simulink model "motor_cont_ctrl0"  (R2018a)
settings: Solver=FixedStepAuto  StartTime=0.0  StopTime=30  RelTol=1e-3
libraries: simulink x1
settings Model: Creator=HuuNgan  LastModifiedBy=HuuNgan

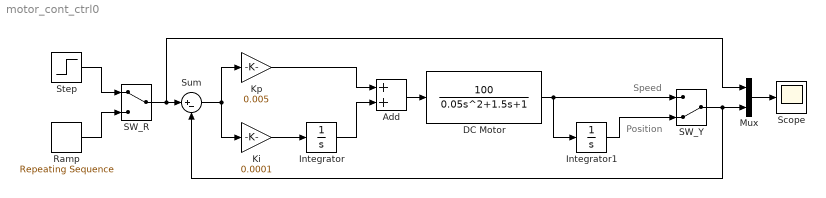
== system motor_cont_ctrl0 ==
  note: Position
  note: Speed
  Add : Sum
  DC Motor : TransferFcn  Numerator=[100]  Denominator=[0.05 1.5 1]
  "Integrator " : Integrator
  Integrator1 : Integrator
  Ki : Gain  Gain=0.0001
  Kp : Gain  Gain=0.005
  Mux : Mux  Inputs=2
  Ramp : simulink/Sources/Repeating Sequence  rep_seq_t=[0 10]  rep_seq_y=[0 800]
  SW_R : ManualSwitch
  SW_Y : ManualSwitch  CurrentSetting=0
  "Scope " : Scope
  "Step " : Step  Time=0  After=1000  SampleTime=0.0001
  Sum : Sum  Inputs=|+-
  wires:
  SW_R/1 -> Mux/1, Sum/1
  Sum/1 -> Ki/1, Kp/1
  Ki/1 -> "Integrator "/1
  Kp/1 -> Add/1
  "Integrator "/1 -> Add/2
  Add/1 -> DC Motor/1
  Integrator1/1 -> SW_Y/2
  DC Motor/1 -> SW_Y/1, Integrator1/1
  "Step "/1 -> SW_R/1
  Ramp/1 -> SW_R/2
  Mux/1 -> "Scope "/1
  SW_Y/1 -> Mux/2, Sum/2
